simulink model "TC_P1_B"  (R2014a)
settings: Solver=ode3  StartTime=0.0  StopTime=20  RelTol=1e-3
libraries: dsparch4 x3, dspmathops x2, commnoisgen2 x1
settings Model: Creator=root  LastModifiedBy=root

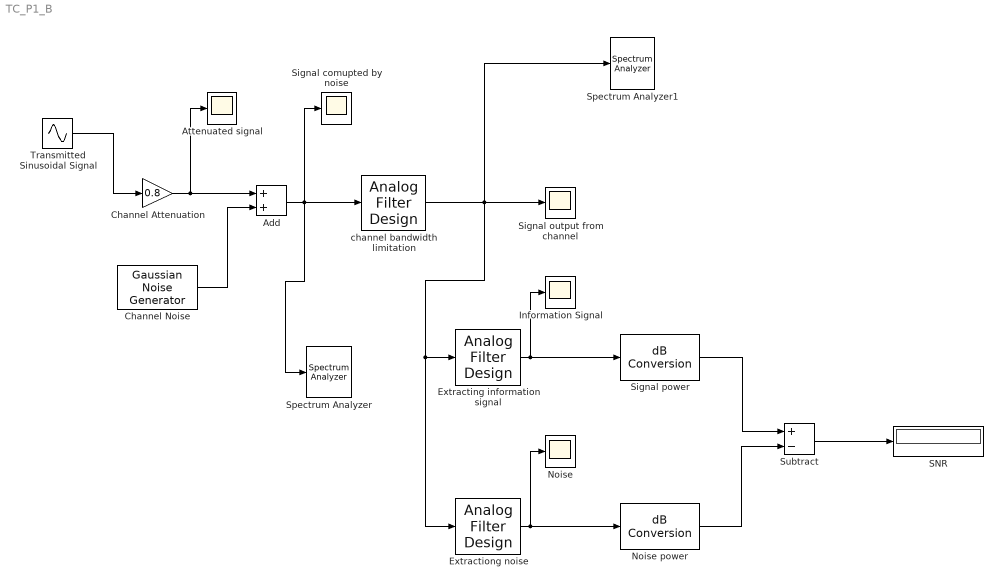
== system TC_P1_B ==
  Add : Sum
  "Attenuated signal " : Scope
      settings: TimeRange=20
  Channel Attenuation : Gain  Gain=0.8
  Channel Noise : commnoisgen2/Gaussian Noise Generator  m=0  d=0.1  s=41  Ts=0.001  frameBased=off  sampPerFrame=1  orient=off  outDataType=double
  Extracting information signal : dsparch4/Analog Filter Design  method=Butterworth  filttype=Bandpass  N=10  Wlo=195  Whi=205  Rp=2  Rs=40
  Extractiong noise : dsparch4/Analog Filter Design  method=Butterworth  filttype=Bandstop  N=10  Wlo=195  Whi=205  Rp=2  Rs=40
  Information Signal : Scope
      settings: SaveName=ScopeData3
  Noise : Scope
      settings: SaveName=ScopeData4
  Noise power : dspmathops/dB Conversion  dBtype=dB  intype=Amplitude  R=1  fuzz=off
  SNR : Display
  Signal comupted by noise : Scope
  Signal output from channel : Scope
      settings: TimeRange=20  SaveName=ScopeData2
  Signal power : dspmathops/dB Conversion  dBtype=dB  intype=Amplitude  R=1  fuzz=off
  Spectrum Analyzer : SpectrumAnalyzer
  Spectrum Analyzer1 : SpectrumAnalyzer
  Subtract : Sum  Inputs=+-
  Transmitted Sinusoidal Signal : Sin  Amplitude=10  Frequency=200  Samples=50  SampleTime=0.001
  channel bandwidth limitation : dsparch4/Analog Filter Design  method=Butterworth  filttype=Lowpass  N=10  Wlo=1000  Whi=80  Rp=2  Rs=40
  wires:
  Channel Noise/1 -> Add/2
  Channel Attenuation/1 -> "Attenuated signal "/1, Add/1
  Transmitted Sinusoidal Signal/1 -> Channel Attenuation/1
  Add/1 -> Spectrum Analyzer/1, channel bandwidth limitation/1, Signal comupted by noise/1
  channel bandwidth limitation/1 -> Spectrum Analyzer1/1, Extractiong noise/1, Extracting information signal/1, Signal output from channel/1
  Extracting information signal/1 -> Signal power/1, Information Signal/1
  Extractiong noise/1 -> Noise power/1, Noise/1
  Signal power/1 -> Subtract/1
  Noise power/1 -> Subtract/2
  Subtract/1 -> SNR/1
